simulink model "corr_hw_test"  (R2012b)
(part 2 of 16)

  ten_Gbe_v4/7 -> Delay32/1(d)
  ten_Gbe_v4/6 -> Delay33/1(d)
  ten_Gbe_v4/10 -> Delay42/1(d)
  Delay44/1(q) -> [dout6]
  unpack3/7(err) -> Delay30/1(d)
  unpack3/8(buf_index) -> Delay34/1(d)
  unpack3/9(sync_chan) -> Delay41/1(d)
  Delay41/1(q) -> [sync_chan6]
  Delay45/1(q) -> [vld6]
  Delay46/1(q) -> [eof6]
  Delay47/1(q) -> [mcnt6]
  Delay43/1(q) -> [ant6]
  Delay31/1(q) -> [flag6]
  Delay30/1(q) -> [err6]
  Delay34/1(q) -> [buf_ind6]
  ten_Gbe_v4/12 -> ten_Gbe_v4/8
  Constant52/1 -> ten_Gbe_v4/7
  Constant55/1 -> ten_Gbe_v4/6
  Constant56/1 -> ten_Gbe_v4/5
  Constant57/1 -> ten_Gbe_v4/4
  Constant58/1 -> ten_Gbe_v4/3
  Constant59/1 -> ten_Gbe_v4/2
  [gbe_rst] -> ten_Gbe_v4/1
  Constant60/1 -> [dout7]
  Constant63/1 -> [vld7]
  Constant47/1 -> [eof7]
  Constant48/1 -> [mcnt7]
  Constant49/1 -> [ant7]
  Constant50/1 -> [err7]
  Constant51/1 -> [sync_chan7]
  Constant53/1 -> [buf_ind7]
  Constant54/1 -> [flag7]
  [ant6] -> pkt_reord3/5(ant)
  [flag6] -> pkt_reord3/6(flag)
  [vld6] -> pkt_reord3/2(valid_in)
  [dout6] -> pkt_reord3/1(din)
  [buf_ind6] -> pkt_reord3/7(buf_index)
  [mcnt6] -> pkt_reord3/4(mcnt)
  [sync_chan6] -> pkt_reord3/8(sync_chan)
  [eof6] -> pkt_reord3/3(eof)
  [dout7] -> pkt_reord3/9(din1)
  [flag7] -> pkt_reord3/14(flag1)
  [eof7] -> pkt_reord3/11(eof1)
  [vld7] -> pkt_reord3/10(valid_in1)
  [mcnt7] -> pkt_reord3/12(mcnt1)
  [ant7] -> pkt_reord3/13(ant1)
  [sync_chan7] -> pkt_reord3/16(sync_chan1)
  [buf_ind7] -> pkt_reord3/15(buf_index1)
  pkt_reord3/1(sync_out) -> [pkt_sync_out3]
  pkt_reord3/2(valid_out) -> [pkt_vld_out3]
  pkt_reord3/3(mcnt_out) -> [pkt_mcnt_out3]
  pkt_reord3/4(dout) -> [pkt_dout3]
  pkt_reord3/7(max_cnt) -> [pkt_max_cnt3]
  [pkt_rd_en3] -> pkt_reord3/18(rd_en)
  [pkt_rd_addr] -> pkt_reord3/19(rd_addr)
  [pkt_cur_window] -> pkt_reord3/20(current_rd_window)
  [ant_id] -> pkt_reord3/17(ant_id)
  [pkt_vld_out2] -> Concat/4, dmux1/4
  [pkt_vld_out1] -> Concat/3, dmux1/3
  [link_id] -> Delay48/1
  [pkt_vld_out3] -> Concat/5, dmux1/5
  [pkt_vld_out0] -> Concat/2, dmux1/2
  Delay48/1 -> Concat/1, dmux1/1
  [pkt_mcnt_out2] -> dmux2/4
  [pkt_mcnt_out1] -> dmux2/3
  [link_id] -> Delay49/1
  [pkt_mcnt_out3] -> dmux2/5
  [pkt_mcnt_out0] -> dmux2/2
  Delay49/1 -> dmux2/1
  [pkt_sync_out2] -> dmux3/4
  [pkt_sync_out1] -> dmux3/3
  [link_id] -> Delay50/1
  [pkt_sync_out3] -> dmux3/5
  [pkt_sync_out0] -> dmux3/2
  Delay50/1 -> dmux3/1
  dmux/1 -> [mux_dout]
  dmux1/1 -> edge_detect/1(in), [mux_vld]
  dmux2/1 -> [mux_mcnt]
  dmux3/1 -> [mux_sync]
  xeng_sp_hdl_uint/2(acc) -> pipeline5/1(d)
  xeng_sp_hdl_uint/1(sync_out) -> pipeline4/1(d)
  xeng_sp_hdl_uint/3(valid) -> pipeline6/1(d)
  xeng_sp_hdl_uint/4(mcnt_out) -> pipeline7/1(d)
  pipeline4/1(q) -> [sync_out]
  pipeline5/1(q) -> [acc_out]
  pipeline6/1(q) -> [vld_out]
  pipeline7/1(q) -> [mcnt_out]
  [mux_dout] -> pipeline9/1(d)
  [mux_vld] -> pipeline8/1(d)
  [mux_mcnt] -> pipeline3/1(d)
  [mux_sync] -> pipeline10/1(d)
  [acc_out] -> vacc1/4(data_in)
  [sync_out] -> vacc1/3(sync_in)
  [vld_out] -> vacc1/5(we)
  [mcnt_out] -> vacc1/6(pcnt_in)
  Convert1/1 -> Concat1/1
  Concat1/1 -> dout/1(din)
  [mcnt_out] -> Convert1/1
  [acc_out] -> Concat1/2
  [vld_out] -> dout/2(we)
  [sync_out] -> dout/3(trig)
  ant_id/1(in_reg) -> Delay51/1(d)
  Delay51/1(q) -> [ant_id]
  Delay52/1(q) -> Slice3/1
  Delay53/1(q) -> Convert/1
  Delay54/1(q) -> Convert2/1
  pkt_reord1/5(lb_last_bad_addr) -> Delay55/1(d)
  pkt_reord1/6(tge_last_bad_addr) -> Delay56/1(d)
  Delay55/1(q) -> Convert4/1
  Delay56/1(q) -> Convert3/1
  pkt_reord2/5(lb_last_bad_addr) -> Delay57/1(d)
  pkt_reord2/6(tge_last_bad_addr) -> Delay58/1(d)
  Delay57/1(q) -> Convert5/1
  Delay58/1(q) -> Convert6/1
  pkt_reord3/5(lb_last_bad_addr) -> Delay59/1(d)
  pkt_reord3/6(tge_last_bad_addr) -> Delay60/1(d)
  Delay59/1(q) -> Convert7/1
  Delay60/1(q) -> Convert8/1
  pipeline3/1(q) -> Convert9/1
  pipeline8/1(q) -> xeng_sp_hdl_uint/3(window_valid), edge_detect1/1(in)
  pipeline9/1(q) -> xeng_sp_hdl_uint/2(ant)
  pipeline10/1(q) -> xeng_sp_hdl_uint/1(sync_in)
  Slice3/1 -> pkt_max_cnt/1(out_reg)
  Convert/1 -> lb_bad_addr0/1(out_reg)
  Convert2/1 -> tge_bad_addr0/1(out_reg)
  Convert3/1 -> tge_bad_addr1/1(out_reg)
  Convert4/1 -> lb_bad_addr1/1(out_reg)
  Convert5/1 -> lb_bad_addr2/1(out_reg)
  Convert6/1 -> tge_bad_addr2/1(out_reg)
  Convert7/1 -> lb_bad_addr3/1(out_reg)
  Convert8/1 -> tge_bad_addr3/1(out_reg)
  Convert9/1 -> xeng_sp_hdl_uint/4(mcnt_in)
  Convert10/1 -> ss_vld/1(din)
  Concat/1 -> Delay61/1
  Delay61/1 -> Convert10/1
  Constant64/1 -> ss_vld/2(we)
  edge_detect/1(out) -> ss_vld/3(trig)
  Counter/1 -> pipeline11/1(d)
  edge_detect1/1(out) -> pipeline12/1(d)
  pipeline11/1(q) -> xeng_inburst_cnt/1(out_reg)
  pipeline12/1(q) -> Counter/2
  [vacc_rst] -> pipeline13/1(d)
  pipeline13/1(q) -> Counter/1
